simulink model "power_monophaseline"  (R2019b)
settings: Solver=FixedStepDiscrete  StartTime=0.0  StopTime=0.1  FixedStep=50e-6  MaxStep=100e-6  RelTol=1e-4
undefined symbols (not defined in the file): Ts
libraries: powerlib x16, artemis x3, op_dpl_lib x1, rtlab x1
settings Model: ARTEMISmethode_block_infos=$$__separator__$$power_monophaseline/SS_Subnetwork_2/ARTEMIS Guide$$__separator__$$  ExtModeTrigMode=oneshot  ExtModeArmWhenConnect=off  ExtModeAutoUpdateStatusClock=off  Creator=MathWorks  LastModifiedBy=Home_PC
settings SolverCC: SolverResetMethod=Robust
settings DataIOCC: SaveFormat=Array  SignalLoggingSaveFormat=ModelDataLogs  SaveOutput=off  SaveTime=off  ReturnWorkspaceOutputs=off  SignalLoggingName=sigsOut
settings OptimizationCC: BlockReduction=off  BooleanDataType=off  ExpressionDepthLimit=2147483647  InitFltsAndDblsToZero=on  EfficientMapNaN2IntZero=off  LifeSpan=inf
settings DebuggingCC: SaveWithParameterizedLinksMsg=none  UnderspecifiedInitializationDetection=Classic  MergeDetectMultiDrivingBlocksExec=none  CheckExecutionContextPreStartOutputMsg=on  CheckExecutionContextRuntimeOutputMsg=on  SignalResolutionControl=TryResolveAllWithWarning  SolverPrmCheckMsg=warning  MultiTaskDSMMsg=warning  MultiTaskCondExecSysMsg=none  SigSpecEnsureSampleTimeMsg=none  IntegerOverflowMsg=none  FcnCallInpInsideContextMsg=warning  StateNameClashWarn=warning  SFUnexpectedBacktrackingDiag=warning  SFNoUnconditionalDefaultTransitionDiag=warning  SFExecutionAtInitializationDiag=none  IntegerSaturationMsg=none  ArithmeticOperatorsInVariantConditions=warning
settings HardwareCC: ProdBitPerPointer=32  ProdBitPerSizeT=32  ProdBitPerPtrDiffT=32  ProdLargestAtomicFloat=None  ProdIntDivRoundTo=Undefined  ProdEndianess=Unspecified  ProdWordSize=32  ProdHWDeviceType=32-bit Generic  TargetUnknown=on
settings ModelReferenceCC: PropagateSignalLabelsOutOfModel=off
settings SFSimCC: SimUseLocalCustomCode=off  CustomCodeUndefinedFunction=UseInterfaceOnly
settings RTWCC: RTWUseLocalCustomCode=off
settings CodeAppCC: StateflowObjectComments=on
settings GRTTargetCC: TargetFcnLib=ansi_tfl_tmw.mat  TargetLangStandard=C89/C90 (ANSI)  GeneratePreprocessorConditionals=Disable all  CombineOutputUpdateFcns=off  GRTInterface=on
settings ConfigComp: CovMetricSettings=dw  CovHtmlReporting=on  CovSaveCumulativeToWorkspaceVar=on  CovSaveSingleToWorkspaceVar=on  CovExternalEMLEnable=off  CovSFcnEnable=off
settings SimscapeCC: SimscapeNormalizeSystem=off

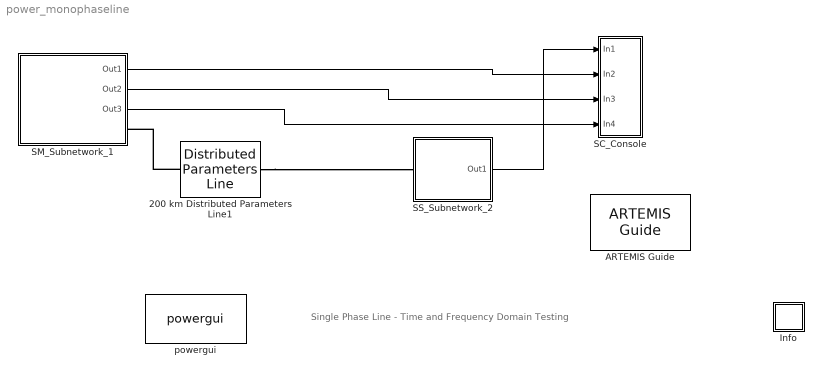
== system power_monophaseline ==
  note: Single Phase Line - Time and Frequency Domain Testing
  200 km Distributed Parameters Line1 : op_dpl_lib/Distributed Parameters Line  SimulationMode=ARTEMIS model  Phases=1  Frequency=60  Resistance=0.0955  Inductance=2.137e-3  Capacitance=12.37e-9  Length=200  Measurements=None
  ARTEMIS Guide : artemis/ARTEMIS/ARTEMIS Guide  Tag=art7.5  Description=New ARTEMiS block v 7.5b (R2015b+)  lock=on  Ts=Ts  ssn=on  opt=art5  dyna=off  nb_perm=4  RT_fullcomp=off  ssn_itvc=off  ssn_ivic=off  ssn_ext=off  ssn_solver=Art5  iter_type=iSWITCH and iMOV only (default)  ssn_ImpulseLoopBlockedStateUpdate=5  ssn_mov_iter_number=5  ssn_switch_iter_number=3  ssn_lu_or_ldlt=LU (more robust)  ssn_nib_type_verify=on  ssn_use_lu=on  ssn_use_ldlt=off  ssn_impulse=on  ssn_quasimpulse=off  ssn_impulse_loop=5  paraExtinctionThy=off  Thy_Impulse=on  dtc=Off  dtc_opt=normal  ao=off  simtype=off  ct_mac=off  lin_mov=off  lsp=[0.001 2]  spike_skip=Disabled  dtc_extra=1  dtc_sws=normal  dtc_pied=0.5  SPSRulesBlock=SPSRules  tre=off  ctmm=off  LF=off  dpl_type=ARTEMiS DPL  rlc_type=off  custom_type=off  para=on  ssn_full_iteration=off  ssn_init_cond=block only
  Info : Subsystem
      settings: OpenFcn=showdemo(bdroot(gcb))
      mask Display: disp('?')
  SC_Console : Subsystem
  SM_Subnetwork_1 : Subsystem
  SS_Subnetwork_2 : Subsystem
  powergui : powerlib/powergui  Priority=2  SimulationMode=Discrete  SampleTime=Ts  frequency=60  Iterations=50  frequencyindice=60  Pbase=100e6  ErrMax=1e-4  UnitsV=kV  UnitsW=MW  buscounter=0  FunctionMessages=off  echomessages=off  EnableUseOfTLC=off  CurrentSourceSwitches=off  DisableSnubberDevices=on  DisableRonSwitches=off  DisableVfSwitches=off  DisplayEquations=off  AutomaticDiscreteSolvers=off  SolverType=Tustin  Interpol=off  ExternalGateDelay=off  methode=off  Ts=0  x0status=blocks  SPID=on  SwTol=0  HookPort=off  NonlinearTolerance=1e-4  nMaxIteration=100  ContinueOnMaxIteration=off  RestoreLinks=warning  ResistiveCurrentMeasurement=off  Frange=0:2:2000  Ylog=on  Xlog=off  ShowGrid=off  save=off  variable=ZData  structure=0  ZoomFFT=on  StartTime=0.0  cycles=1  DisplayStyle=off  fundamental=60  FreqAxis=off  MaxFrequency=1000  frequencyindicesteady=1  RmsSteady=1  display=on
      settings: SourceProductName=Simscape Electrical
  wires:
  SS_Subnetwork_2/1(Out1) -> SC_Console/1(In1)
  SM_Subnetwork_1/1(Out1) -> SC_Console/2(In2)
  SM_Subnetwork_1/2(Out2) -> SC_Console/3(In3)
  SM_Subnetwork_1/3(Out3) -> SC_Console/4(In4)
  connections:
  200 km Distributed Parameters Line1/LConn1 -- SM_Subnetwork_1/RConn1
  200 km Distributed Parameters Line1/RConn1 -- SS_Subnetwork_2/LConn1

== system power_monophaseline/Info ==

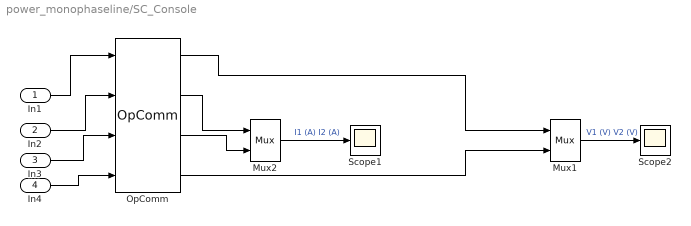
== system power_monophaseline/SC_Console ==
  In1 : Inport
  In2 : Inport  Port=2
  In3 : Inport  Port=3
  In4 : Inport  Port=4
  Mux1 : Mux  Inputs=2
  Mux2 : Mux  Inputs=2
  OpComm : rtlab/OpComm  nbport=4  groupe_acq=1  subsys_rate=0  st=0  Synchronization=on  Interpolation=on  Threshold=1.0  Missed_Data=off  Sim_Time=off  Samples=off  dynSigOut=off  from_console=0  warning_done=off  writeOpCommFile=off  Offset=off
      settings: SourceProductName=RT-LAB
  Scope1 : Scope
  Scope2 : Scope
  wires:
  In4/1 -> OpComm/4
  Mux2/1 -> Scope1/1  "I1 (A) I2 (A)"
  Mux1/1 -> Scope2/1  "V1 (V) V2 (V)"
  In1/1 -> OpComm/1
  OpComm/1 -> Mux1/1
  In2/1 -> OpComm/2
  OpComm/2 -> Mux2/1
  In3/1 -> OpComm/3
  OpComm/3 -> Mux2/2
  OpComm/4 -> Mux1/2

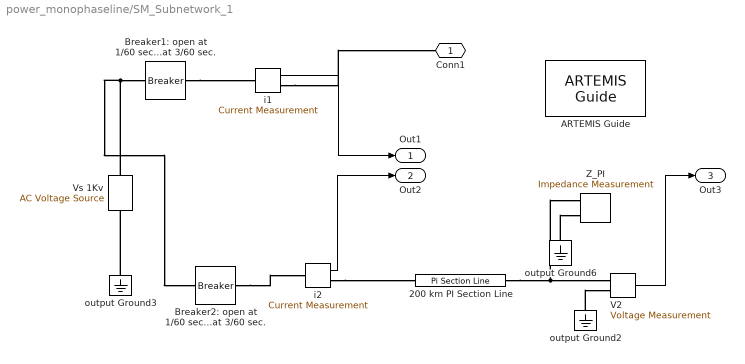
== system power_monophaseline/SM_Subnetwork_1 ==
  200 km PI Section Line : powerlib/Elements/Pi Section Line  LConnTagsString=__new0  RConnTagsString=__new0  Frequency=60  Resistance=0.0955  Inductance=2.137e-03  Capacitance=12.37e-09  Length=200  PiSections=2  Measurements=None
      settings: AttributesFormatString=\n  SourceProductName=Simscape Electrical  SourceProductBaseCode=PS
  ARTEMIS Guide : artemis/ARTEMIS/ARTEMIS Guide  Tag=art7.5  Description=New ARTEMiS block v 7.5b (R2015b+)  lock=on  Ts=Ts  ssn=on  opt=art5  dyna=off  nb_perm=4  RT_fullcomp=off  ssn_itvc=off  ssn_ivic=off  ssn_ext=off  ssn_solver=Art5  iter_type=iSWITCH and iMOV only (default)  ssn_ImpulseLoopBlockedStateUpdate=5  ssn_mov_iter_number=5  ssn_switch_iter_number=3  ssn_lu_or_ldlt=LU (more robust)  ssn_nib_type_verify=on  ssn_use_lu=on  ssn_use_ldlt=off  ssn_impulse=on  ssn_quasimpulse=off  ssn_impulse_loop=5  paraExtinctionThy=off  Thy_Impulse=on  dtc=Off  dtc_opt=normal  ao=off  simtype=off  ct_mac=off  lin_mov=off  lsp=[0.001 2]  spike_skip=Disabled  dtc_extra=1  dtc_sws=normal  dtc_pied=0.5  SPSRulesBlock=SPSRules  tre=off  ctmm=off  LF=off  dpl_type=ARTEMiS DPL  rlc_type=off  custom_type=off  para=on  ssn_full_iteration=off  ssn_init_cond=block only
  Breaker1: open at 1/60 sec. close at 3/60 sec. : powerlib/Elements/Breaker  InitialState=1  SwitchingTimes="[ 1/60  3/60 ]"  External=off  BreakerResistance=0.1  SnubberResistance=inf  SnubberCapacitance=0  Measurements=None  MoreParameters=off  NoBreakLoop=off
      settings: AttributesFormatString=\n  SourceProductName=Simscape Electrical
  Breaker2: open at 1/60 sec. close at 3/60 sec. : powerlib/Elements/Breaker  InitialState=1  SwitchingTimes="[ 1/60  3/60 ]"  External=off  BreakerResistance=0.1  SnubberResistance=inf  SnubberCapacitance=0  Measurements=None  MoreParameters=off  NoBreakLoop=off
      settings: AttributesFormatString=\n  SourceProductName=Simscape Electrical
  V2 : powerlib/Measurements/Voltage Measurement  Tag=PoWeRsYsTeMmEaSuReMeNt  PhasorSimulation=off  OutputType=Magnitude  PSBequivalent=0
      settings: SourceProductName=Simscape Electrical
  Vs 1Kv : powerlib/Electrical Sources/AC Voltage Source  Description=source block  Amplitude=1e3  Phase=0  Frequency=60  SampleTime=0  Measurements=None  BusType=swing  Pref=10e3  Qref=0  Qmin=-inf  Qmax=+inf
      settings: AttributesFormatString=\n  SourceProductName=Simscape Electrical
  Z_PI : powerlib/Measurements/Impedance Measurement  LConnTagsString=+|-  Factor=1
      settings: AttributesFormatString=\n  SourceProductName=Simscape Electrical  SourceProductBaseCode=PS
  i1 : powerlib/Measurements/Current Measurement  Tag=PoWeRsYsTeMmEaSuReMeNt  PhasorSimulation=off  OutputType=Magnitude  PSBequivalent=0
      settings: SourceProductName=Simscape Electrical
  i2 : powerlib/Measurements/Current Measurement  Tag=PoWeRsYsTeMmEaSuReMeNt  PhasorSimulation=off  OutputType=Magnitude  PSBequivalent=0
      settings: SourceProductName=Simscape Electrical
  output Ground2 : powerlib/Elements/Ground  LConnTagsString=a
      settings: SourceProductName=Simscape Electrical
  output Ground3 : powerlib/Elements/Ground  LConnTagsString=a
      settings: SourceProductName=Simscape Electrical
  output Ground6 : powerlib/Elements/Ground  LConnTagsString=a
      settings: SourceProductName=Simscape Electrical
  Conn1 : PMIOPort  Side=Right
  Out1 : Outport
  Out2 : Outport  Port=2
  Out3 : Outport  Port=3
  wires:
  i2/1 -> Out2/1
  i1/1 -> Out1/1
  V2/1 -> Out3/1
  connections:
  Breaker2: open at 1/60 sec. close at 3/60 sec./RConn1 -- i2/LConn1
  Breaker1: open at 1/60 sec. close at 3/60 sec./RConn1 -- i1/LConn1
  output Ground3/LConn1 -- Vs 1Kv/LConn1
  Vs 1Kv/RConn1 -- Breaker1: open at 1/60 sec. close at 3/60 sec./LConn1 -- Breaker2: open at 1/60 sec. close at 3/60 sec./LConn1
  200 km PI Section Line/RConn1 -- V2/LConn1 -- Z_PI/LConn1
  output Ground6/LConn1 -- Z_PI/LConn2
  i2/RConn1 -- 200 km PI Section Line/LConn1
  output Ground2/LConn1 -- V2/LConn2
  i1/RConn1 -- Conn1/RConn1

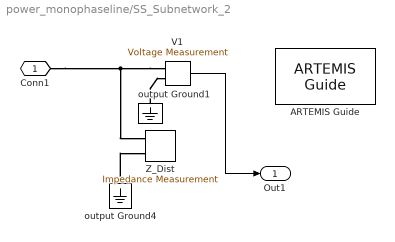
== system power_monophaseline/SS_Subnetwork_2 ==
  ARTEMIS Guide : artemis/ARTEMIS/ARTEMIS Guide  Tag=art7.5  Description=New ARTEMiS block v 7.5b (R2015b+)  lock=on  Ts=Ts  ssn=on  opt=art5  dyna=off  nb_perm=4  RT_fullcomp=off  ssn_itvc=off  ssn_ivic=off  ssn_ext=off  ssn_solver=Art5  iter_type=iSWITCH and iMOV only (default)  ssn_ImpulseLoopBlockedStateUpdate=5  ssn_mov_iter_number=5  ssn_switch_iter_number=3  ssn_lu_or_ldlt=LU (more robust)  ssn_nib_type_verify=on  ssn_use_lu=on  ssn_use_ldlt=off  ssn_impulse=on  ssn_quasimpulse=off  ssn_impulse_loop=5  paraExtinctionThy=off  Thy_Impulse=on  dtc=Off  dtc_opt=normal  ao=off  simtype=off  ct_mac=off  lin_mov=off  lsp=[0.001 2]  spike_skip=Disabled  dtc_extra=1  dtc_sws=normal  dtc_pied=0.5  SPSRulesBlock=SPSRules  tre=off  ctmm=off  LF=off  dpl_type=ARTEMiS DPL  rlc_type=off  custom_type=off  para=on  ssn_full_iteration=off  ssn_init_cond=block only
  V1 : powerlib/Measurements/Voltage Measurement  Tag=PoWeRsYsTeMmEaSuReMeNt  PhasorSimulation=off  OutputType=Magnitude  PSBequivalent=0
      settings: SourceProductName=Simscape Electrical
  Z_Dist : powerlib/Measurements/Impedance Measurement  LConnTagsString=+|-  Factor=1
      settings: AttributesFormatString=\n  SourceProductName=Simscape Electrical  SourceProductBaseCode=PS
  output Ground1 : powerlib/Elements/Ground  LConnTagsString=a
      settings: SourceProductName=Simscape Electrical
  output Ground4 : powerlib/Elements/Ground  LConnTagsString=a
      settings: SourceProductName=Simscape Electrical
  Conn1 : PMIOPort  Side=Left
  Out1 : Outport
  wires:
  V1/1 -> Out1/1
  connections:
  output Ground4/LConn1 -- Z_Dist/LConn2
  V1/LConn1 -- Conn1/RConn1 -- Z_Dist/LConn1
  output Ground1/LConn1 -- V1/LConn2
